simulink model "codesAnalyseKasami"  (R2012b)
settings: Solver=ode45  StartTime=0.0  StopTime=10.0  RelTol=1e-3
undefined symbols (not defined in the file or in its folder): get
libraries: dspstat3 x2, commseqgen2 x2, commutil2 x2, dspsnks4 x2
settings Model: Creator=mcaceres  LastModifiedBy=mcaceres

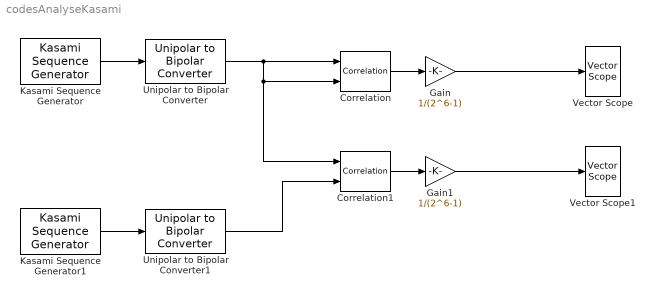
== system codesAnalyseKasami ==
  Correlation : dspstat3/Correlation  domain=Time  outputDataTypeStr=Inherit: Same as accumulator  outputLastDataTypeStr=Inherit: Same as accumulator  outputMin=[]  outputMax=[]  roundingMode=Floor  overflowMode=off
  Correlation1 : dspstat3/Correlation  domain=Time  outputDataTypeStr=Inherit: Same as accumulator  outputLastDataTypeStr=Inherit: Same as accumulator  outputMin=[]  outputMax=[]  roundingMode=Floor  overflowMode=off
  Gain : Gain  Gain=1/(2^6-1)
  Gain1 : Gain  Gain=1/(2^6-1)
  Kasami Sequence Generator : commseqgen2/Kasami Sequence Generator  genPoly=[1 0 0 0 0 1 1]  iniState=[0 0 0 0 0 1]  codeIdx=5  shift=0  outVarSiz=off  maxOutSizeMode=Dialog parameter  maxOutSize=[10 1]  ts=10^-6/(2^6-1)  frameBased=on  sampPerFrame=63  reset=off  outDataType=double
  Kasami Sequence Generator1 : commseqgen2/Kasami Sequence Generator  genPoly=[1 0 0 0 0 1 1]  iniState=[0 0 0 0 0 1]  codeIdx=1  shift=0  outVarSiz=off  maxOutSizeMode=Dialog parameter  maxOutSize=[10 1]  ts=1  frameBased=off  sampPerFrame=1  reset=off  outDataType=double
  Unipolar to Bipolar Converter : commutil2/Unipolar to Bipolar Converter  M=2  polarity=Positive  dataType=Inherit via internal rule
  Unipolar to Bipolar Converter1 : commutil2/Unipolar to Bipolar Converter  M=2  polarity=Positive  dataType=Inherit via internal rule
  Vector Scope : dspsnks4/Vector Scope  ScopeProperties=on  Domain=Time  HorizSpan=1  DisplayProperties=off  AxisGrid=on  Memory=off  FrameNumber=on  AxisLegend=off  AxisZoom=off  OpenScopeAtSimStart=on  OpenScopeImmediately=off  FigPos=get(0,'defaultfigureposition')  AxisProperties=off  XUnits=Hertz  XRange=[0...Fs/2]  InheritXIncr=on  XIncr=1  XLabel=Time  XLimit=Auto  XMin=0  XMax=1  XStart=0  YUnits=dB  YLabel=Amplitude  LineProperties=off  XAxisParamsVer=6.9
      settings: YMin=-10  YMax=10
  Vector Scope1 : dspsnks4/Vector Scope  ScopeProperties=on  Domain=Time  HorizSpan=1  DisplayProperties=off  AxisGrid=on  Memory=off  FrameNumber=on  AxisLegend=off  AxisZoom=off  OpenScopeAtSimStart=on  OpenScopeImmediately=off  FigPos=get(0,'defaultfigureposition')  AxisProperties=off  XUnits=Hertz  XRange=[0...Fs/2]  InheritXIncr=on  XIncr=1  XLabel=Time  XLimit=Auto  XMin=0  XMax=1  XStart=0  YUnits=dB  YLabel=Amplitude  LineProperties=off  XAxisParamsVer=6.9
      settings: YMin=-10  YMax=10
  wires:
  Correlation/1 -> Gain/1
  Correlation1/1 -> Gain1/1
  Gain/1 -> Vector Scope/1
  Gain1/1 -> Vector Scope1/1
  Kasami Sequence Generator/1 -> Unipolar to Bipolar Converter/1
  Unipolar to Bipolar Converter/1 -> Correlation1/1, Correlation/2, Correlation/1
  Unipolar to Bipolar Converter1/1 -> Correlation1/2
  Kasami Sequence Generator1/1 -> Unipolar to Bipolar Converter1/1
